simulink model "pwmDriver"  (R2021a)
settings: Solver=FixedStepAuto  StartTime=0.0  StopTime=10.0  RelTol=1e-3
undefined symbols (not defined in the file): fpwm
libraries: simulink x1
settings Model: Creator=Z634594  LastModifiedBy=Z634594

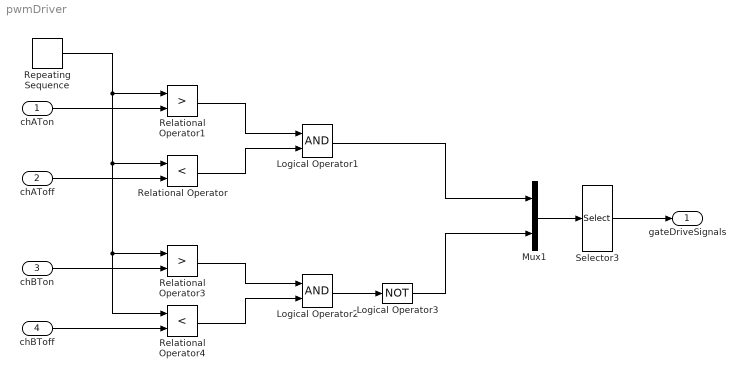
== system pwmDriver ==
  chATon : Inport  PortDimensions=3
  chAToff : Inport  Port=2  PortDimensions=3
  chBTon : Inport  Port=3  PortDimensions=3
  chBToff : Inport  Port=4  PortDimensions=3
  Logical Operator1 : Logic  AllPortsSameDT=off  OutDataTypeStr=boolean
  Logical Operator2 : Logic  AllPortsSameDT=off  OutDataTypeStr=boolean
  Logical Operator3 : Logic  Operator=NOT  AllPortsSameDT=off  OutDataTypeStr=boolean
  Mux1 : Mux  Inputs=2
  Relational Operator : RelationalOperator  Operator=<  OutDataTypeStr=boolean  RndMeth=Simplest
  Relational Operator1 : RelationalOperator  Operator=>  OutDataTypeStr=boolean  RndMeth=Simplest
  Relational Operator3 : RelationalOperator  Operator=>  OutDataTypeStr=boolean  RndMeth=Simplest
  Relational Operator4 : RelationalOperator  Operator=<  OutDataTypeStr=boolean  RndMeth=Simplest
  Repeating Sequence : simulink/Sources/Repeating Sequence  rep_seq_t=[0 1/fpwm]  rep_seq_y=[0 1/fpwm]
  Selector3 : Selector  InputPortWidth=6  IndexOptions=Index vector (dialog)  Indices=[1 4 2 5 3 6]  OutputSizes=1
  gateDriveSignals : Outport
  wires:
  chAToff/1 -> Relational Operator/2
  chBToff/1 -> Relational Operator4/2
  Selector3/1 -> gateDriveSignals/1
  Repeating Sequence/1 -> Relational Operator4/1, Relational Operator3/1, Relational Operator/1, Relational Operator1/1
  chATon/1 -> Relational Operator1/2
  Logical Operator2/1 -> Logical Operator3/1
  Relational Operator3/1 -> Logical Operator2/1
  Logical Operator1/1 -> Mux1/1
  chBTon/1 -> Relational Operator3/2
  Relational Operator4/1 -> Logical Operator2/2
  Logical Operator3/1 -> Mux1/2
  Mux1/1 -> Selector3/1
  Relational Operator1/1 -> Logical Operator1/1
  Relational Operator/1 -> Logical Operator1/2
